simulink model "InClarkPark_Test"  (R2025b)
settings: Solver=VariableStepAuto  StartTime=0.0  StopTime=10.0  RelTol=1e-3
libraries: MyPMSMLibrary x1
settings Model: Creator=jff_1  LastModifiedBy=jff_1

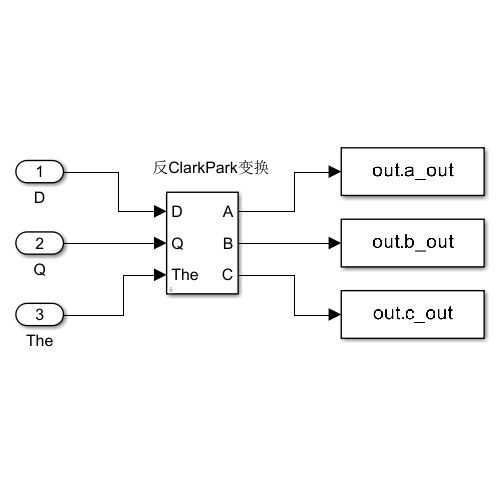
[thumbnail: Simulink's stored preview of the top-level diagram]
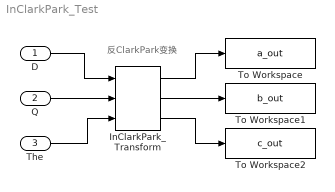
== system InClarkPark_Test ==
  note: 反ClarkPark变换
  D : Inport
  Q : Inport  Port=2
  The : Inport  Port=3
  InClarkPark_Transform : MyPMSMLibrary/Transforms/InClarkPark_Transform
  To Workspace : ToWorkspace  VariableName=a_out  SaveFormat=Timeseries  SampleTime=-1
  To Workspace1 : ToWorkspace  VariableName=b_out  SaveFormat=Timeseries  SampleTime=-1
  To Workspace2 : ToWorkspace  VariableName=c_out  SaveFormat=Timeseries  SampleTime=-1
  wires:
  D/1 -> InClarkPark_Transform/1
  Q/1 -> InClarkPark_Transform/2
  The/1 -> InClarkPark_Transform/3
  InClarkPark_Transform/1 -> To Workspace/1
  InClarkPark_Transform/2 -> To Workspace1/1
  InClarkPark_Transform/3 -> To Workspace2/1
